simulink model "BrakingSystemPlant"  (Simulink 8.5)
settings: Solver=ode45  StartTime=0.0  StopTime=20  RelTol=1e-3
values from neighbouring files (symbols this model uses):
  mpod = 441.    (= 441)    [allthesimulations.m]    (also in brakingTrajectory.m = 320; hoverengine_dynamics_vs_track_oscillation.m = 350; simParameters.m = 360)
  xdot0 = xdot(n)    [Trajectory.m]    (also in brakingTrajectory.m = 120)
settings Model: Creator=MrPiccolo  LastModifiedBy=MrPiccolo
settings DataIOCC: SignalLoggingSaveFormat=Dataset
settings OptimizationCC: ExpressionDepthLimit=128
settings DebuggingCC: UnderspecifiedInitializationDetection=Simplified  MergeDetectMultiDrivingBlocksExec=error  FcnCallInpInsideContextMsg=EnableAllAsError  StateNameClashWarn=none
settings GRTTargetCC: CombineOutputUpdateFcns=on  GRTInterface=off

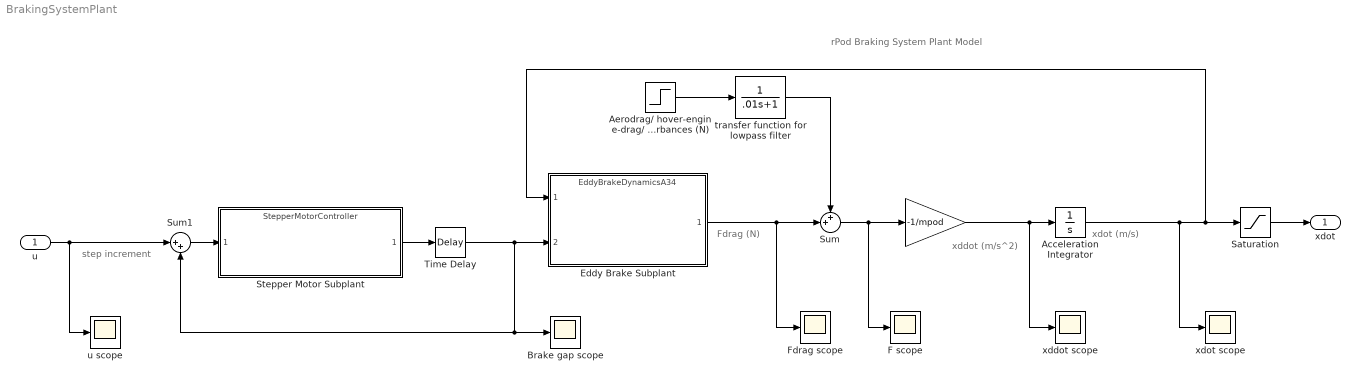
== system BrakingSystemPlant ==
  note: Fdrag (N)
  note: xddot (m/s^2)
  note: xdot (m/s)
  note: rPod Braking System
      | Plant Model
  note: step increment
  u : Inport
  " " : Gain  Gain=-1/mpod
  Acceleration Integrator : Integrator  InitialCondition=xdot0
  Aerodrag/ hover-engine-drag/ Disturbances (N) : Step  After=0  SampleTime=0
  Brake gap scope : Scope
      settings: TimeRange=20  YMin=0  YMax=25  SaveName=ScopeData6
  Eddy Brake Subplant : ModelReference  ModelNameDialog=EddyBrakeDynamicsA34.mdl  SimulationMode=Normal  ModelReferenceVersion=1.5  CopyOfModelName=EddyBrakeDynamicsA34.mdl  DefaultDataLogging=on
  F scope : Scope
      settings: SaveName=ScopeData5
  Fdrag scope : Scope
  Saturation : Saturate  UpperLimit=300  LowerLimit=0
  Stepper Motor Subplant : ModelReference  ModelNameDialog=StepperMotorController.mdl  SimulationMode=Normal  ModelReferenceVersion=1.72  CopyOfModelName=StepperMotorController.mdl  DefaultDataLogging=on
  Sum : Sum  Inputs=++|
  Sum1 : Sum  Inputs=|++
  Time Delay : TransportDelay  DelayTime=.01
  transfer function for lowpass filter : TransferFcn  Denominator=[.01 1]
  u scope : Scope
      settings: YMin=2.09908  YMax=25.3146
  xddot scope : Scope
      settings: SaveName=ScopeData4
  xdot scope : Scope
      settings: TimeRange=40  YMin=2.0991  YMax=25.3146  SaveName=ScopeData2
  xdot : Outport
  wires:
  " "/1 -> xddot scope/1, Acceleration Integrator/1
  Stepper Motor Subplant/1 -> Time Delay/1
  Aerodrag/ hover-engine-drag/ Disturbances (N)/1 -> transfer function for lowpass filter/1
  Acceleration Integrator/1 -> Eddy Brake Subplant/1, Saturation/1, xdot scope/1
  u/1 -> Sum1/1, u scope/1
  Eddy Brake Subplant/1 -> Fdrag scope/1, Sum/2
  Saturation/1 -> xdot/1
  Sum/1 -> F scope/1, " "/1
  transfer function for lowpass filter/1 -> Sum/1
  Sum1/1 -> Stepper Motor Subplant/1
  Time Delay/1 -> Eddy Brake Subplant/2, Brake gap scope/1, Sum1/2
